simulink library "Gimbal_Lib"  (R2020a)
settings: Solver=VariableStepAuto  StartTime=0.0  StopTime=10.0  RelTol=1e-3
values from neighbouring files (symbols this model uses):
  degs_per_step = 0.025    [Main_mat.m]
  pulse_len = 100    [Main_mat.m]
  speed_factor = 38000    [Main_mat.m]
libraries: $bdroot x3, simulink x1
settings Model: Creator=idan  LastModifiedBy=idan

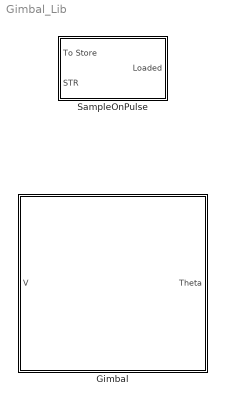
== system Gimbal_Lib ==
  Gimbal : Subsystem  mask{NullSpeedDelay=0}
      mask prompts: NullSpeedDelay "Null Speed Delay"
      mask TypeOptions NullSpeedDelay: Null Speed Delay/Value
  SampleOnPulse : Subsystem

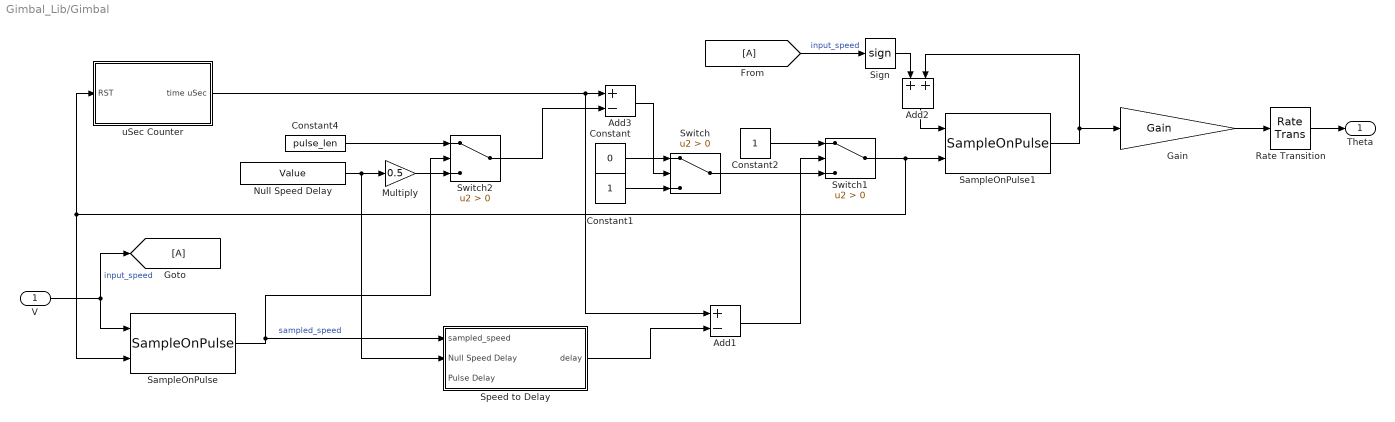
== system Gimbal_Lib/Gimbal ==
  V : Inport
  Add1 : Sum  Inputs=+-
  Add2 : Sum
  Add3 : Sum  Inputs=+-
  Constant : Constant  Value=0
  Constant1 : Constant
  Constant2 : Constant
  Constant4 : Constant  Value=pulse_len
  Gain : Gain  Gain=Gain  ParamDataTypeStr=Inherit: Inherit from 'Gain'  mask{Gain=degs_per_step}
      mask prompts: Gain "Simulink:blkprm_prompts:GainGain"
      mask TypeOptions Gain: Gain
      mask DialogControl Gain Prompt: Gain:
  Multiply : Gain  Gain=0.5
  Null Speed Delay : Constant  Value=Value  mask{Value=NullSpeedDelay}
      mask prompts: Value "Simulink:blkprm_prompts:ConstConstValue"
      mask TypeOptions Value: Value
      mask DialogControl Value Prompt: Constant value:
  Rate Transition : RateTransition  OutPortSampleTime=1/100
  SampleOnPulse : $bdroot/SampleOnPulse  SystemSampleTime=-1  Latency=0  AutoFrameSizeCalculation=off
  SampleOnPulse1 : $bdroot/SampleOnPulse  SystemSampleTime=-1  Latency=0  AutoFrameSizeCalculation=off
  Sign : Signum
  Speed to Delay : Subsystem
  Switch : Switch  Criteria=u2 > Threshold
  Switch1 : Switch  Criteria=u2 > Threshold
  Switch2 : Switch  Criteria=u2 > Threshold
  uSec Counter : Subsystem
  Theta : Outport
  wires:
  Constant/1 -> Switch/1
  Constant1/1 -> Switch/3
  Switch/1 -> Switch1/3
  Constant2/1 -> Switch1/1
  Switch1/1 -> SampleOnPulse1/2, uSec Counter/1(RST), SampleOnPulse/2
  V/1 -> [A], SampleOnPulse/1  "input_speed"
  Add1/1 -> Switch1/2
  [A] -> Sign/1  "input_speed"
  Add2/1 -> SampleOnPulse1/1
  Sign/1 -> Add2/1
  uSec Counter/1(time uSec) -> Add3/1, Add1/1
  SampleOnPulse/1 -> Speed to Delay/1(sampled_speed), Switch2/2  "sampled_speed"
  Speed to Delay/1(delay) -> Add1/2
  Constant4/1 -> Switch2/1
  Switch2/1 -> Add3/2
  Add3/1 -> Switch/2
  SampleOnPulse1/1 -> Add2/2, Gain/1
  Gain/1 -> Rate Transition/1
  Rate Transition/1 -> Theta/1
  Null Speed Delay/1 -> Speed to Delay/2(Null Speed Delay), Multiply/1
  Multiply/1 -> Switch2/3

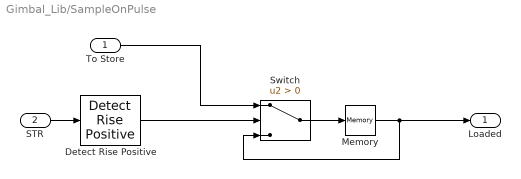
== system Gimbal_Lib/SampleOnPulse ==
  To Store : Inport
  STR : Inport  Port=2
  Detect Rise Positive : simulink/Logic and Bit Operations/Detect Rise Positive  vinit=0  OutDataTypeStr=uint8
  Memory : Memory  InheritSampleTime=on
  Switch : Switch  Criteria=u2 > Threshold
  Loaded : Outport
  wires:
  STR/1 -> Detect Rise Positive/1
  Detect Rise Positive/1 -> Switch/2
  Memory/1 -> Loaded/1, Switch/3
  Switch/1 -> Memory/1
  To Store/1 -> Switch/1

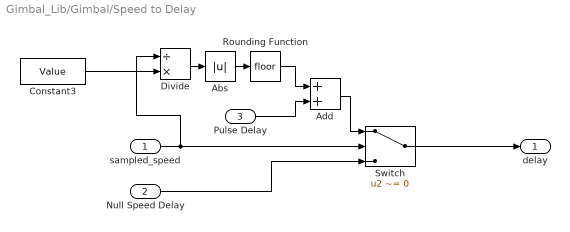
== system Gimbal_Lib/Gimbal/Speed to Delay ==
  sampled_speed : Inport
  Null Speed Delay : Inport  Port=2
  Pulse Delay : Inport  Port=3
  Abs : Abs
  Add : Sum
  Constant3 : Constant  Value=Value  mask{Value=speed_factor}
      mask prompts: Value "Simulink:blkprm_prompts:ConstConstValue"
      mask TypeOptions Value: Value
      mask DialogControl Value Prompt: Constant value:
  Divide : Product  Inputs=/*
  Rounding Function : Rounding
  Switch : Switch  Criteria=u2 ~= 0
  delay : Outport
  wires:
  Divide/1 -> Abs/1
  Abs/1 -> Rounding Function/1
  sampled_speed/1 -> Divide/1, Switch/2
  Switch/1 -> delay/1
  Constant3/1 -> Divide/2
  Rounding Function/1 -> Add/1
  Pulse Delay/1 -> Add/2
  Add/1 -> Switch/1
  Null Speed Delay/1 -> Switch/3

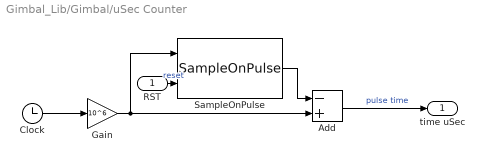
== system Gimbal_Lib/Gimbal/uSec Counter ==
  RST : Inport
  Add : Sum  Inputs=-+
  Clock : Clock
  Gain : Gain  Gain=10^6
  SampleOnPulse : $bdroot/SampleOnPulse  SystemSampleTime=-1  Latency=0  AutoFrameSizeCalculation=off
  time uSec : Outport
  wires:
  SampleOnPulse/1 -> Add/1
  Clock/1 -> Gain/1
  Gain/1 -> Add/2, SampleOnPulse/1
  Add/1 -> time uSec/1  "pulse time"
  RST/1 -> SampleOnPulse/2  "reset"
